simulink model "modulator"  (R2017b)
settings: Solver=FixedStepDiscrete  StartTime=0.0  StopTime=10  RelTol=1e-3
libraries: dspsrcs4 x2, hdlsllib x1
settings Model: DataTypeOverride=Off  Creator=jake  LastModifiedBy=mw
settings DataIOCC: SaveOutput=off  SaveTime=off
settings OptimizationCC: BlockReduction=off  ConditionallyExecuteInputs=off  DefaultParameterBehavior=Inlined
settings DebuggingCC: AlgebraicLoopMsg=error  SingleTaskRateTransMsg=error  StrictBusMsg=ErrorOnBusTreatedAsVector
settings HardwareCC: ProdBitPerPointer=32  ProdBitPerSizeT=32  ProdBitPerPtrDiffT=32  ProdLargestAtomicFloat=None  ProdIntDivRoundTo=Undefined  ProdEndianess=Unspecified  ProdWordSize=32  ProdHWDeviceType=ASIC/FPGA->ASIC/FPGA  ProdEqTarget=off
settings CodeAppCC: StateflowObjectComments=on
settings GRTTargetCC: TargetLangStandard=C89/C90 (ANSI)

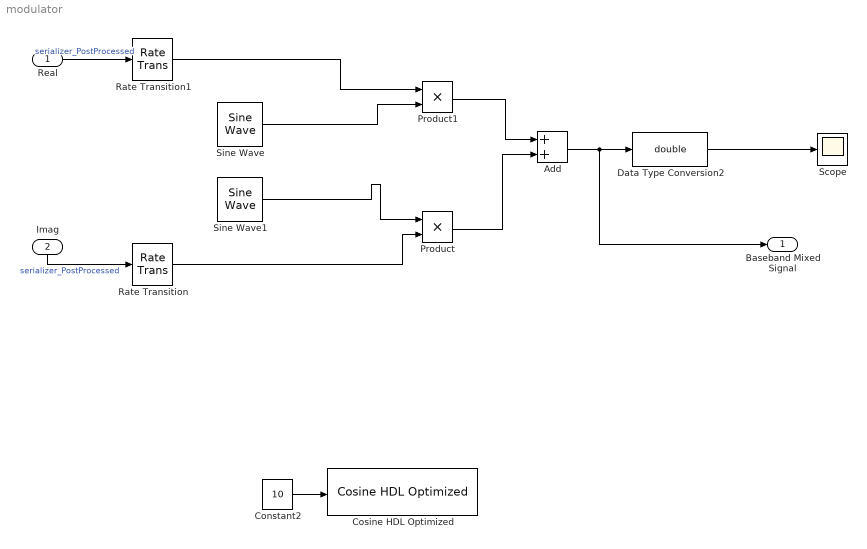
== system modulator ==
  Real : Inport  OutDataTypeStr=fixdt(1,20,13)  PortDimensions=1  SampleTime=[0.0001,0]
  Imag : Inport  Port=2  OutDataTypeStr=fixdt(1,20,13)  PortDimensions=1  SampleTime=[0.0001,0]
  Add : Sum
  Constant2 : Constant  Value=10  VectorParams1D=off  OutDataTypeStr=int8
  Cosine HDL Optimized : hdlsllib/Lookup Tables/Cosine HDL Optimized  OutputFormula=sin(2*pi*u) and cos(2*pi*u)  NumDataPoints=64  TableDataTypeStr=fixdt(1,16,0)  SimulateLUTROMDelay=off
      settings: SourceProductName=HDL Coder  SourceProductBaseCode=HD
  Data Type Conversion2 : DataTypeConversion  OutDataTypeStr=double
  Product : Product
  Product1 : Product
  Rate Transition : RateTransition
  Rate Transition1 : RateTransition
  Scope : Scope
  Sine Wave : dspsrcs4/Sine Wave  Amplitude=1  Frequency=1000  Phase=0  SampleMode=Discrete  OutComplex=Real  CompMethod=Table lookup  TableSize=Speed  SampleTime=1/10000  SamplesPerFrame=1  ResetState=Restart at time zero  OutputFrames=off  dataType=Fixed-point  wordLen=16  udDataType=sfix(16)  fracBitsMode=User-defined  numFracBits=14  OutDataTypeStr=fixdt(1,16,14)  LastOutDataTypeStr=fixdt(1,16,14)
  Sine Wave1 : dspsrcs4/Sine Wave  Amplitude=1  Frequency=1000  Phase=pi/2  SampleMode=Discrete  OutComplex=Real  CompMethod=Table lookup  TableSize=Speed  SampleTime=1/10000  SamplesPerFrame=1  ResetState=Restart at time zero  OutputFrames=off  dataType=Fixed-point  wordLen=16  udDataType=sfix(16)  fracBitsMode=User-defined  numFracBits=14  OutDataTypeStr=fixdt(1,16,14)  LastOutDataTypeStr=fixdt(1,16,14)
  Baseband Mixed Signal : Outport  OutDataTypeStr=fixdt(1,37,27)  PortDimensions=[1 1]  SampleTime=[0.0001,0]
  wires:
  Data Type Conversion2/1 -> Scope/1
  Rate Transition1/1 -> Product1/1
  Rate Transition/1 -> Product/2
  Product1/1 -> Add/1
  Product/1 -> Add/2
  Add/1 -> Data Type Conversion2/1, Baseband Mixed Signal/1
  Sine Wave/1 -> Product1/2
  Sine Wave1/1 -> Product/1
  Constant2/1 -> Cosine HDL Optimized/1
  Real/1 -> Rate Transition1/1  "serializer_PostProcessed"
  Imag/1 -> Rate Transition/1  "serializer_PostProcessed"
